simulink model "Mandana"  (R2015a)
settings: Solver=ode45  StartTime=0.0  StopTime=20  RelTol=1e-3
libraries: fuzblock x1
settings Model: Creator=ROJO  LastModifiedBy=ROJO

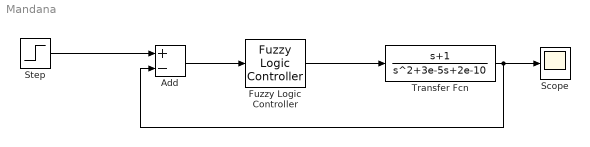
== system Mandana ==
  Add : Sum  Inputs=+-
  Fuzzy Logic Controller : fuzblock/Fuzzy Logic  Controller  fis=FUZZY_MANDANA
  Scope : Scope
  Step : Step  After=5  SampleTime=0
  Transfer Fcn : TransferFcn  Numerator=[1 1]  Denominator=[1 3e-5 2e-10]
  wires:
  Fuzzy Logic Controller/1 -> Transfer Fcn/1
  Add/1 -> Fuzzy Logic Controller/1
  Step/1 -> Add/1
  Transfer Fcn/1 -> Add/2, Scope/1
